simulink model "Quad_Model_X"  (R2015b)
settings: Solver=ode45  StartTime=0.0  StopTime=10.0  RelTol=1e-3
values from neighbouring files (symbols this model uses):
  Ixx = 1.395e-05    [mdl_quadrotor.m]
  Iyy = 1.395e-05    [mdl_quadrotor.m]
  Izz = 2.173e-05    [mdl_quadrotor.m]
undefined symbols (not defined in the file or in its folder): quad
settings Model: Creator=Carlos  LastModifiedBy=carlosluis
settings DataIOCC: SaveFormat=Array
settings DebuggingCC: UnderspecifiedInitializationDetection=Classic  MergeDetectMultiDrivingBlocksExec=none  SolverPrmCheckMsg=warning  StateNameClashWarn=warning
settings HardwareCC: ProdBitPerPointer=32  ProdLargestAtomicFloat=None  ProdIntDivRoundTo=Undefined  ProdEndianess=Unspecified  ProdWordSize=32  ProdHWDeviceType=32-bit Generic
settings GRTTargetCC: GeneratePreprocessorConditionals=Disable all
settings ConfigComp: CovModelRefEnable=Off

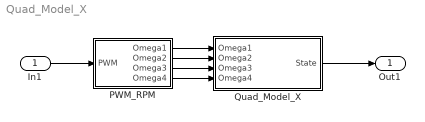
== system Quad_Model_X ==
  In1 : Inport
  PWM_RPM : Subsystem
  Quad_Model_X : Subsystem
  Out1 : Outport
  wires:
  Quad_Model_X/1(State) -> Out1/1
  PWM_RPM/1(Omega1) -> Quad_Model_X/1(Omega1)
  PWM_RPM/2(Omega2) -> Quad_Model_X/2(Omega2)
  PWM_RPM/3(Omega3) -> Quad_Model_X/3(Omega3)
  PWM_RPM/4(Omega4) -> Quad_Model_X/4(Omega4)
  In1/1 -> PWM_RPM/1(PWM)

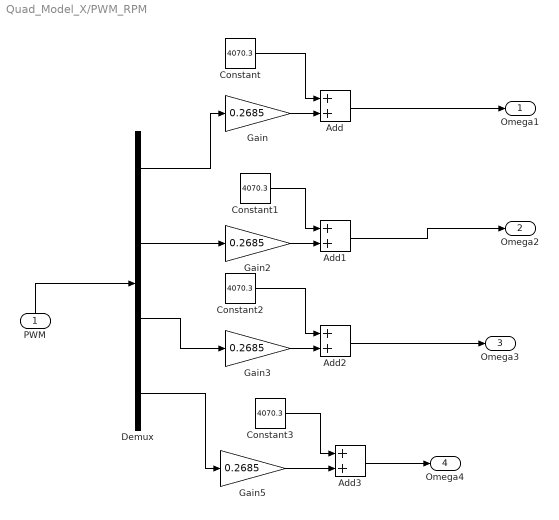
== system Quad_Model_X/PWM_RPM ==
  PWM : Inport
  Add{,1..3} (4 alike) : Sum
  Constant{,1..3} (4 alike) : Constant  Value=4070.3
  Demux : Demux
  Gain{,2..3,5} (4 alike) : Gain  Gain=0.2685
  Omega1 : Outport
  Omega2 : Outport  Port=2
  Omega3 : Outport  Port=3
  Omega4 : Outport  Port=4
  wires:
  Gain/1 -> Add/2
  Demux/1 -> Gain/1
  Demux/4 -> Gain5/1
  Gain5/1 -> Add3/2
  Constant3/1 -> Add3/1
  Add3/1 -> Omega4/1
  Constant1/1 -> Add1/1
  Gain2/1 -> Add1/2
  Demux/2 -> Gain2/1
  Add1/1 -> Omega2/1
  PWM/1 -> Demux/1
  Add/1 -> Omega1/1
  Add2/1 -> Omega3/1
  Demux/3 -> Gain3/1
  Constant2/1 -> Add2/1
  Gain3/1 -> Add2/2
  Constant/1 -> Add/1

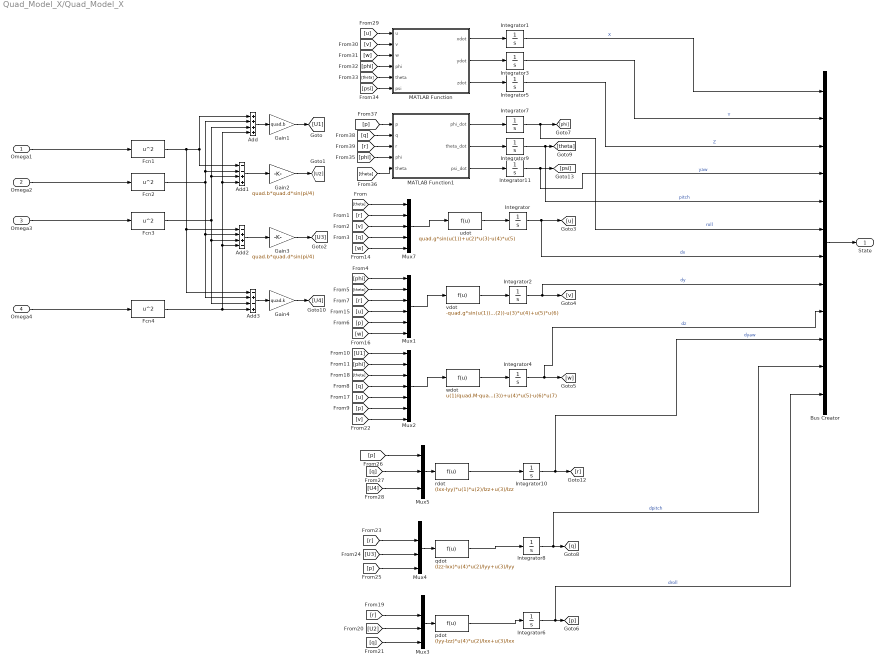
== system Quad_Model_X/Quad_Model_X ==
  Omega1 : Inport
  Omega2 : Inport  Port=2
  Omega3 : Inport  Port=3
  Omega4 : Inport  Port=4
  Add : Sum  Inputs=++++
  Add1 : Sum  Inputs=--++
  Add2 : Sum  Inputs=-++-
  Add3 : Sum  Inputs=-+-+
  Bus Creator : BusCreator  Inputs=12
  Fcn{1..4} (4 alike) : Fcn  Expr=u^2
  Gain1 : Gain  Gain=quad.b
  Gain2 : Gain  Gain=quad.b*quad.d*sin(pi/4)
  Gain3 : Gain  Gain=quad.b*quad.d*sin(pi/4)
  Gain4 : Gain  Gain=quad.k
  Integrator{,1..11} (12 alike) : Integrator
  MATLAB Function : MATLAB Function  TreatAsAtomicUnit=on
  MATLAB Function1 : MATLAB Function  TreatAsAtomicUnit=on
  Mux1 : Mux  Inputs=6
  Mux2 : Mux  Inputs=7
  Mux3 : Mux
  Mux4 : Mux
  Mux5 : Mux  Inputs=3
  Mux7 : Mux  Inputs=5
  pdot : Fcn  Expr=(Iyy-Izz)*u(4)*u(2)/Ixx+u(3)/Ixx
  qdot : Fcn  Expr=(Izz-Ixx)*u(4)*u(2)/Iyy+u(3)/Iyy
  rdot : Fcn  Expr=(Ixx-Iyy)*u(1)*u(2)/Izz+u(3)/Izz
  "udot " : Fcn  Expr=quad.g*sin(u(1))+u(2)*u(3)-u(4)*u(5)
  "vdot " : Fcn  Expr=-quad.g*sin(u(1))*cos(u(2))-u(3)*u(4)+u(5)*u(6)
  "wdot " : Fcn  Expr=u(1)/quad.M-quad.g*cos(u(2))*cos(u(3))+u(4)*u(5)-u(6)*u(7)
  State : Outport
  wires:
  Integrator5/1 -> Bus Creator/3  "Z"
  Integrator3/1 -> Bus Creator/2  "Y"
  Integrator1/1 -> Bus Creator/1  "X"
  [r] -> MATLAB Function1/3(r)
  [q] -> MATLAB Function1/2(q)
  [p] -> MATLAB Function1/1(p)
  [psi] -> MATLAB Function/6(psi)
  Integrator7/1 -> [phi], Bus Creator/6  "roll"
  Integrator9/1 -> [theta], Bus Creator/5  "pitch"
  Integrator11/1 -> [psi], Bus Creator/4  "yaw"
  MATLAB Function1/3(psi_dot) -> Integrator11/1
  MATLAB Function1/2(theta_dot) -> Integrator9/1
  MATLAB Function1/1(phi_dot) -> Integrator7/1
  MATLAB Function/3(zdot) -> Integrator5/1
  MATLAB Function/2(ydot) -> Integrator3/1
  MATLAB Function/1(xdot) -> Integrator1/1
  [theta] -> MATLAB Function1/5(theta)
  [phi] -> MATLAB Function1/4(phi)
  [theta] -> MATLAB Function/5(theta)
  [phi] -> MATLAB Function/4(phi)
  [w] -> MATLAB Function/3(w)
  [v] -> MATLAB Function/2(v)
  [u] -> MATLAB Function/1(u)
  [v] -> Mux2/7
  [p] -> Mux2/6
  [u] -> Mux2/5
  [U1] -> Mux2/1
  [q] -> Mux2/4
  [theta] -> Mux2/3
  Mux2/1 -> "wdot "/1
  [phi] -> Mux2/2
  [w] -> Mux1/6
  [p] -> Mux1/5
  [phi] -> Mux1/1
  [u] -> Mux1/4
  [r] -> Mux1/3
  Mux1/1 -> "vdot "/1
  [theta] -> Mux1/2
  [w] -> Mux7/5
  pdot/1 -> Integrator6/1
  qdot/1 -> Integrator8/1
  rdot/1 -> Integrator10/1
  Gain1/1 -> [U1]
  Fcn4/1 -> Add/4, Add1/4, Add2/4, Add3/4
  Fcn3/1 -> Add1/3, Add/3, Add2/3, Add3/3
  Fcn2/1 -> Add2/2, Add3/2, Add1/2, Add/2
  Fcn1/1 -> Add/1, Add1/1, Add2/1, Add3/1
  [r] -> Mux3/2
  [q] -> Mux3/4
  [q] -> Mux5/2
  Mux4/1 -> qdot/1
  [U2] -> Mux3/3
  Integrator4/1 -> [w], Bus Creator/9  "dz"
  "wdot "/1 -> Integrator4/1
  Bus Creator/1 -> State/1
  [p] -> Mux4/4
  Mux3/1 -> pdot/1
  Integrator10/1 -> [r], Bus Creator/10  "dyaw"
  Integrator6/1 -> [p], Bus Creator/12  "droll"
  [r] -> Mux4/2
  [U4] -> Mux5/3
  [p] -> Mux5/1
  Mux5/1 -> rdot/1
  [U3] -> Mux4/3
  Integrator8/1 -> [q], Bus Creator/11  "dpitch"
  Add1/1 -> Gain2/1
  Add/1 -> Gain1/1
  Omega2/1 -> Fcn2/1
  [theta] -> Mux7/1
  Integrator2/1 -> [v], Bus Creator/8  "dy"
  "vdot "/1 -> Integrator2/1
  Omega1/1 -> Fcn1/1
  [q] -> Mux7/4
  Add2/1 -> Gain3/1
  Gain2/1 -> [U2]
  [v] -> Mux7/3
  Gain4/1 -> [U4]
  Integrator/1 -> [u], Bus Creator/7  "dx"
  "udot "/1 -> Integrator/1
  Mux7/1 -> "udot "/1
  [r] -> Mux7/2
  Omega3/1 -> Fcn3/1
  Omega4/1 -> Fcn4/1
  Add3/1 -> Gain4/1
  Gain3/1 -> [U3]

== matlab function Quad_Model_X/MATLAB Function ==
  data: u input; xdot output; v input; w input; phi input; theta input; psi input; ydot output; zdot output
function [xdot,ydot,zdot] = fcn(u,v,w,phi,theta,psi)

xdot= u*cos(theta)*cos(psi)+v*(sin(phi)*sin(theta)*cos(psi)-cos(phi)*sin(psi))+w*(cos(phi)*sin(theta)*cos(psi)+sin(phi)*sin(psi));

ydot= u*cos(theta)*sin(psi)+v*(sin(phi)*sin(theta)*sin(psi)+cos(phi)*cos(psi))+w*(cos(phi)*sin(theta)*sin(psi)-sin(phi)*cos(psi));

zdot = -u*sin(theta)+v*sin(phi)*cos(theta)+w*cos(phi)*cos(theta);
end

== matlab function Quad_Model_X/MATLAB Function1 ==
  data: p input; phi_dot output; q input; r input; phi input; theta input; theta_dot output; psi_dot output
function [phi_dot,theta_dot,psi_dot] = fcn(p,q,r,phi,theta)
phi_dot = p+q*tan(theta)*sin(phi)+r*tan(theta)*cos(phi);
theta_dot = q*cos(phi)-r*sin(phi);
psi_dot = q*sin(phi)/cos(theta)+r*cos(phi)/cos(theta);
end
